simulink model "Simulink"  (R2024b)
settings: Solver=FixedStepAuto  StartTime=0.0  StopTime=tf_sim  FixedStep=dt/time_scale  MaxStep=dt/100  RelTol=1e-3
values from neighbouring files (symbols this model uses):
  A_ref = zeros(nx,nx,N_ref)    [Main.m]
  b_bar = repmat(b_tilde,N,1)    [Main.m]
  B_ref = zeros(nx,nu,N_ref)    [Main.m]
  d = 0.1    [Main.m]
  dt = tf_ref/N_ref    [Main.m]
  H_ter = Xf.A    [Main.m]
  h_ter = Xf.b    [Main.m]
  IC = x_ref(1,:)'+e0    [Main.m]
  IC_obs = [IC_obs_state; IC_obs_d]    [Main.m]
  N = 20    [Main.m]
  nu = size(u_ref,2)    [Main.m]
  nx = size(x_ref,2)    [Main.m]
  Q_obs = blkdiag(Qw,Qp)    [Main.m]
  R_obs = diag([1 1 1])    [Main.m]
  time_scale = 100    [Main.m]
  Ub_lb = repmat(u_min,N_ref,1)-Umat2Uvect(u_ref)    [Main.m]
  Ub_ub = repmat(u_max,N_ref,1)-Umat2Uvect(u_ref)    [Main.m]
undefined symbols (not defined in the file or in its folder): H_sim, h_sim, S_sim, T_sim, x0
settings Model: Creator=nicvi  LastModifiedBy=nicvi

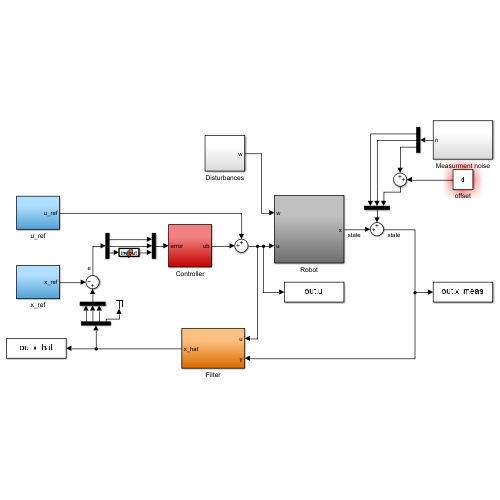
[thumbnail: Simulink's stored preview of the top-level diagram]
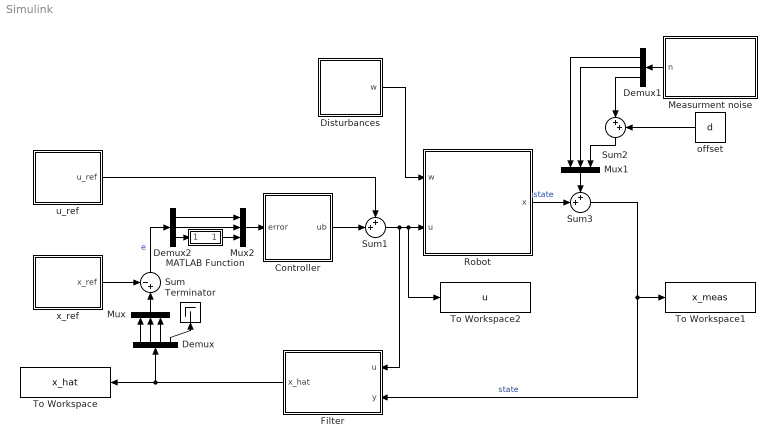
== system Simulink ==
  Controller : Subsystem
  Demux : Demux
  Demux1 : Demux  Outputs=3
  Demux2 : Demux  Outputs=3
  Disturbances : Subsystem
  Filter : Subsystem
  MATLAB Function : MATLAB Function  TreatAsAtomicUnit=on
  Measurment noise : Subsystem
  Mux : Mux  Inputs=3
  Mux1 : Mux  Inputs=3
  Mux2 : Mux  Inputs=3
  Robot : Subsystem
  Sum : Sum  Inputs=-+|
  Sum1 : Sum  Inputs=++|
  Sum2 : Sum  Inputs=|++
  Sum3 : Sum  Inputs=++|
  Terminator : Terminator
  To Workspace : ToWorkspace  VariableName=x_hat  SampleTime=-1
  To Workspace1 : ToWorkspace  VariableName=x_meas  SampleTime=-1
  To Workspace2 : ToWorkspace  VariableName=u  SampleTime=dt/time_scale
  offset : Constant  Value=d
  u_ref : Subsystem
  x_ref : Subsystem
  wires:
  x_ref/1(x_ref) -> Sum/1
  Controller/1(ub) -> Sum1/2
  u_ref/1(u_ref) -> Sum1/1
  Sum/1 -> Demux2/1  "e"
  Sum3/1 -> Filter/2(y), To Workspace1/1  "state"
  Sum1/1 -> Filter/1(u), Robot/2(u), To Workspace2/1
  Robot/1(x) -> Sum3/2  "state"
  Disturbances/1(w) -> Robot/1(w)
  Filter/1(x_hat) -> To Workspace/1, Demux/1
  Demux/1 -> Mux/1
  Demux/4 -> Terminator/1
  Demux/2 -> Mux/2
  Demux/3 -> Mux/3
  Mux/1 -> Sum/2
  Measurment noise/1(n) -> Demux1/1
  offset/1 -> Sum2/2
  Demux1/3 -> Sum2/1
  Demux1/1 -> Mux1/1
  Demux1/2 -> Mux1/2
  Sum2/1 -> Mux1/3
  Mux1/1 -> Sum3/1
  Demux2/3 -> MATLAB Function/1(in)
  MATLAB Function/1(out) -> Mux2/3
  Demux2/1 -> Mux2/1
  Demux2/2 -> Mux2/2
  Mux2/1 -> Controller/1(error)

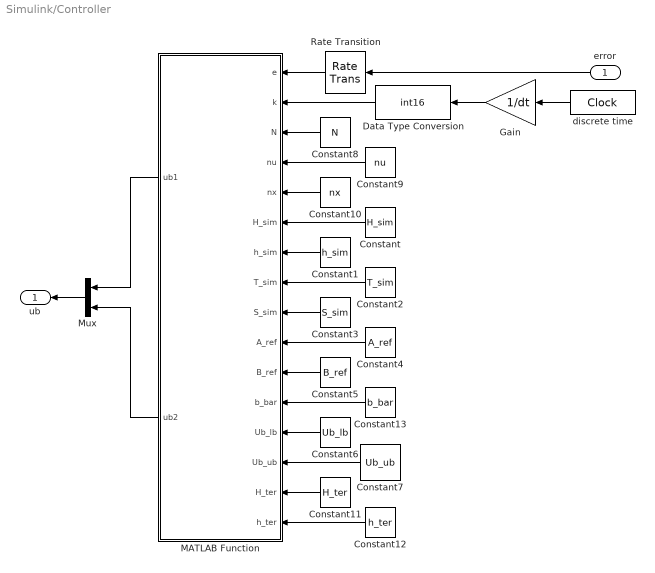
== system Simulink/Controller ==
  error : Inport
  Constant : Constant  Value=H_sim
  Constant1 : Constant  Value=h_sim
  Constant10 : Constant  Value=nx
  Constant11 : Constant  Value=H_ter
  Constant12 : Constant  Value=h_ter
  Constant13 : Constant  Value=b_bar
  Constant2 : Constant  Value=T_sim
  Constant3 : Constant  Value=S_sim
  Constant4 : Constant  Value=A_ref
  Constant5 : Constant  Value=B_ref
  Constant6 : Constant  Value=Ub_lb
  Constant7 : Constant  Value=Ub_ub
  Constant8 : Constant  Value=N
  Constant9 : Constant  Value=nu
  Data Type Conversion : DataTypeConversion  OutDataTypeStr=int16  SaturateOnIntegerOverflow=off  RndMeth=Floor
  Gain : Gain  Gain=1/dt
  MATLAB Function : MATLAB Function  TreatAsAtomicUnit=on
  Mux : Mux  Inputs=2
  Rate Transition : RateTransition  OutPortSampleTime=dt
  discrete time : DigitalClock  SampleTime=dt
  ub : Outport
  wires:
  Constant4/1 -> MATLAB Function/10(A_ref)
  Data Type Conversion/1 -> MATLAB Function/2(k)
  discrete time/1 -> Gain/1
  Gain/1 -> Data Type Conversion/1
  Rate Transition/1 -> MATLAB Function/1(e)
  Constant/1 -> MATLAB Function/6(H_sim)
  Constant10/1 -> MATLAB Function/5(nx)
  Constant11/1 -> MATLAB Function/15(H_ter)
  Constant13/1 -> MATLAB Function/12(b_bar)
  Constant5/1 -> MATLAB Function/11(B_ref)
  Constant3/1 -> MATLAB Function/9(S_sim)
  Constant6/1 -> MATLAB Function/13(Ub_lb)
  Constant9/1 -> MATLAB Function/4(nu)
  Constant7/1 -> MATLAB Function/14(Ub_ub)
  Constant12/1 -> MATLAB Function/16(h_ter)
  Constant8/1 -> MATLAB Function/3(N)
  Constant1/1 -> MATLAB Function/7(h_sim)
  Constant2/1 -> MATLAB Function/8(T_sim)
  error/1 -> Rate Transition/1
  MATLAB Function/1(ub1) -> Mux/1
  MATLAB Function/2(ub2) -> Mux/2
  Mux/1 -> ub/1

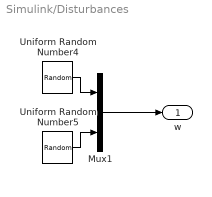
== system Simulink/Disturbances ==
  Mux1 : Mux  Inputs=2
  Uniform Random Number4 : UniformRandomNumber  Minimum=-0.01  Maximum=0.01  SampleTime=0.01
  Uniform Random Number5 : UniformRandomNumber  Minimum=-0.01  Maximum=0.01  SampleTime=0.01
  w : Outport
  wires:
  Uniform Random Number4/1 -> Mux1/1
  Uniform Random Number5/1 -> Mux1/2
  Mux1/1 -> w/1

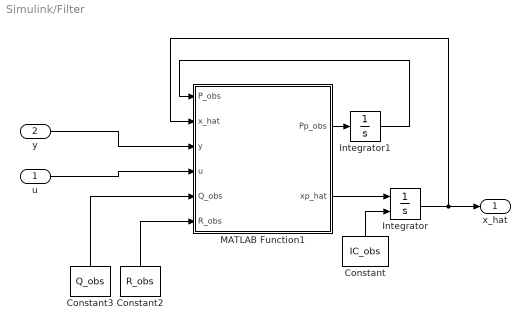
== system Simulink/Filter ==
  u : Inport
  y : Inport  Port=2
  Constant : Constant  Value=IC_obs
  Constant2 : Constant  Value=R_obs
  Constant3 : Constant  Value=Q_obs
  Integrator : Integrator  InitialConditionSource=external
  Integrator1 : Integrator  InitialCondition=zeros(nx+1,nx+1)
  MATLAB Function1 : MATLAB Function  TreatAsAtomicUnit=on
  x_hat : Outport
  wires:
  MATLAB Function1/2(xp_hat) -> Integrator/1
  Constant/1 -> Integrator/2
  Integrator/1 -> MATLAB Function1/2(x_hat), x_hat/1
  MATLAB Function1/1(Pp_obs) -> Integrator1/1
  Integrator1/1 -> MATLAB Function1/1(P_obs)
  u/1 -> MATLAB Function1/4(u)
  Constant3/1 -> MATLAB Function1/5(Q_obs)
  Constant2/1 -> MATLAB Function1/6(R_obs)
  y/1 -> MATLAB Function1/3(y)

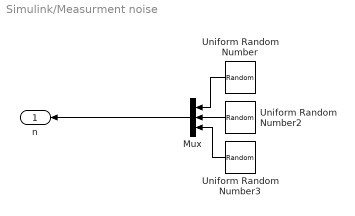
== system Simulink/Measurment noise ==
  Mux : Mux  Inputs=3
  Uniform Random Number : UniformRandomNumber  Minimum=-0.1  Maximum=0.1  SampleTime=0.01
  Uniform Random Number2 : UniformRandomNumber  Minimum=-0.1  Maximum=0.1  SampleTime=0.01
  Uniform Random Number3 : UniformRandomNumber  Minimum=-0.01  Maximum=0.01  SampleTime=0.01
  n : Outport
  wires:
  Uniform Random Number3/1 -> Mux/3
  Uniform Random Number/1 -> Mux/1
  Uniform Random Number2/1 -> Mux/2
  Mux/1 -> n/1

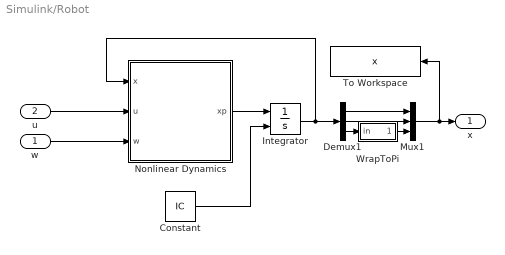
== system Simulink/Robot ==
  w : Inport
  u : Inport  Port=2
  Constant : Constant  Value=IC
  Demux1 : Demux  Outputs=3
  Integrator : Integrator  InitialConditionSource=external  InitialCondition=x0
  Mux1 : Mux  Inputs=3
  Nonlinear Dynamics : MATLAB Function  TreatAsAtomicUnit=on
  To Workspace : ToWorkspace  VariableName=x  SampleTime=dt/time_scale
  WrapToPi : MATLAB Function  TreatAsAtomicUnit=on
  x : Outport
  wires:
  Nonlinear Dynamics/1(xp) -> Integrator/1
  u/1 -> Nonlinear Dynamics/2(u)
  Constant/1 -> Integrator/2
  w/1 -> Nonlinear Dynamics/3(w)
  Demux1/3 -> WrapToPi/1(in)
  Integrator/1 -> Demux1/1, Nonlinear Dynamics/1(x)
  Demux1/1 -> Mux1/1
  WrapToPi/1(out) -> Mux1/3
  Demux1/2 -> Mux1/2
  Mux1/1 -> To Workspace/1, x/1

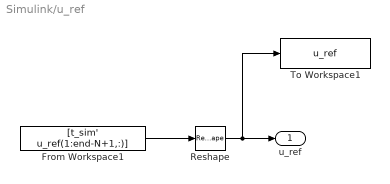
== system Simulink/u_ref ==
  From Workspace1 : FromWorkspace  VariableName="[t_sim'  u_ref(1:end-N+1,:)]"  SampleTime=dt
  Reshape : Reshape  OutputDimensionality=Column vector (2-D)
  To Workspace1 : ToWorkspace  VariableName=u_ref  SampleTime=dt/time_scale
  u_ref : Outport
  wires:
  From Workspace1/1 -> Reshape/1
  Reshape/1 -> To Workspace1/1, u_ref/1

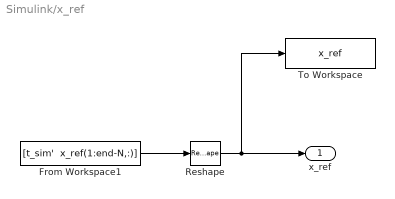
== system Simulink/x_ref ==
  From Workspace1 : FromWorkspace  VariableName="[t_sim'  x_ref(1:end-N,:)]"  SampleTime=dt
  Reshape : Reshape  OutputDimensionality=Column vector (2-D)
  To Workspace : ToWorkspace  VariableName=x_ref  SampleTime=dt/time_scale
  x_ref : Outport
  wires:
  From Workspace1/1 -> Reshape/1
  Reshape/1 -> To Workspace/1, x_ref/1

== matlab function Simulink/Controller/MATLAB Function ==
  data: e input; k input; ub1 output; N input; nu input; ub2 output; nx input; H_sim input; h_sim input; T_sim input; S_sim input; A_ref input; B_ref input; b_bar input; Ub_lb input; Ub_ub input; H_ter input; h_ter input
function [ub1,ub2]=MPC(e,k,N,nu,nx,H_sim,h_sim,T_sim,S_sim,A_ref,B_ref,b_bar,Ub_lb,Ub_ub,H_ter,h_ter)

k=k+1;
options=optimoptions('quadprog','Algorithm','active-set');

% Extract current matrices
H=H_sim(:,:,k);
h=h_sim(:,:,k);
T=T_sim(:,:,k);
S=S_sim(:,:,k);
A_ref_pred=A_ref(:,:,k:k+N-1);
B_ref_pred=B_ref(:,:,k:k+N-1);

% Generate constraints matrices
U_LB=Ub_lb((k-1)*nu+1:(k-1+N)*nu);  % estract lower bounds for ub in the current prediction horizon (input constraints)
U_UB=Ub_ub((k-1)*nu+1:(k-1+N)*nu);  % estract upper bounds for ub in the current prediction horizon (input constraints)
A_bar=zeros(2*N*nx,N*nx);                                                                     % generate matrices for inequality constraints ("state" (error) constraints)
B_bar=zeros(2*N*nx,N*nu);                                                                     % ...
for ii=1:N                                                                                    % ...
    A_bar(2*nx*(ii-1)+1:2*nx*ii,nx*(ii-1)+1:nx*ii)=[A_ref_pred(:,:,ii); -A_ref_pred(:,:,ii)]; % ...
    B_bar(2*nx*(ii-1)+1:2*nx*ii,nu*(ii-1)+1:nu*ii)=[B_ref_pred(:,:,ii); -B_ref_pred(:,:,ii)]; % ...
end                                                                                           % ...
A_ineq1=A_bar*S(1:end-nx,:)+B_bar;                                                            % ...
b_ineq1=b_bar-A_bar*T(1:end-nx,:)*e;                                                          % ...
A_ineq2=H_ter*S(end-nx+1:end,:);          % terminal constraint for the final error e(N) in the current horizon
b_ineq2=h_ter-H_ter*T(end-nx+1:end,:)*e;  % ...
A_ineq=[A_ineq1; A_ineq2];   % "total" inequality constraints
b_ineq=[b_ineq1; b_ineq2];   % ...

% quadprog solver for optimization
U0=(U_LB+U_UB)/2;
Ub_opt=quadprog(H,h*e,A_ineq,b_ineq,[],[],U_LB,U_UB,U0,options);

% Extract first control step
ub=Ub_opt(1:nu)';
ub1=ub(1);
ub2=ub(2);

end

== matlab function Simulink/Robot/Nonlinear Dynamics ==
  data: x input; u input; xp output; w input
function xp =Robot(x,u,w)

xp=zeros(3,1);
xp(1)=(u(1)+w(1))*cos(x(3));
xp(2)=(u(1)+w(1))*sin(x(3));
xp(3)=u(2)+w(2);

end

== matlab function Simulink/Filter/MATLAB Function1 ==
  data: P_obs input; Pp_obs output; x_hat input; y input; xp_hat output; u input; Q_obs input; R_obs input
function [Pp_obs,xp_hat]=EKF(P_obs,x_hat,y,u,Q_obs,R_obs)

nx=3;  % states
nw=2;  % input disturbance
nd=1;  % measurment offset

% Extended system model

f=@(x,u) [u(1)*cos(x(3));      % nonlinear extended model of the system - dynamics
          u(1)*sin(x(3));
               u(2)     
                0       ];  

h=@(x) [x(1) x(2) x(3)+x(4)]'; % nonlinear extended model of the system - output equation

% Linearisation around the extimated state

Aa=zeros(nx+nd,nx+nd);       % Aa = dfdx|x_hat,u
Aa(1,3)=-u(1)*sin(x_hat(3));
Aa(2,3)=u(1)*cos(x_hat(3));

Ca=[eye(nx) [0 0 1]'];       % Ca = dhdx|x_hat,u

La=zeros(nx+nd,nw+nd);       % La = dfdw|x_hat,u
La(1,1)=cos(x_hat(3));
La(2,1)=sin(x_hat(3));
La(3,2)=1;
La(4,3)=1;

Ma=eye(nx);                  % Ma = dhdn|x_hat,u

% Differential Riccati equation (P_obs is the (nx,nx) Riccati matrix)

Pp_obs=Aa*P_obs+P_obs*Aa'+La*Q_obs*La'-P_obs*Ca'*inv(Ma*R_obs*Ma')*Ca*P_obs;

% Kalman gain equation

K_obs=P_obs*Ca'*inv(R_obs);

% Filter equation

xp_hat=f(x_hat,u)+K_obs*(y-h(x_hat));

end

== matlab function Simulink/Robot/WrapToPi ==
  data: in input; out output
function out = fcn(in)

out=wrapToPi(in);

== matlab function Simulink/MATLAB Function ==
  data: in input; out output
function out = fcn(in)

out=mod(in+pi,2*pi)-pi;
